simulink model "slx4"  (R2023b)
settings: Solver=ode4  StartTime=0.0  StopTime=100  FixedStep=0.01  RelTol=1e-3
values from neighbouring files (symbols this model uses):
  epsilon = sqrt((1/A_Dq)-1)    [m8.m]
  l1 = 2    [pendelPlot.m]
  l2 = 4    [pendelPlot.m]
  m1 = lsim(F1,x,t)    [m8.m]
  m2 = lsim(F2,x,t)    [m8.m]
undefined symbols (not defined in the file or in its folder): g
libraries: realtime_pacer_lib x1
settings Model: Creator=user  LastModifiedBy=user

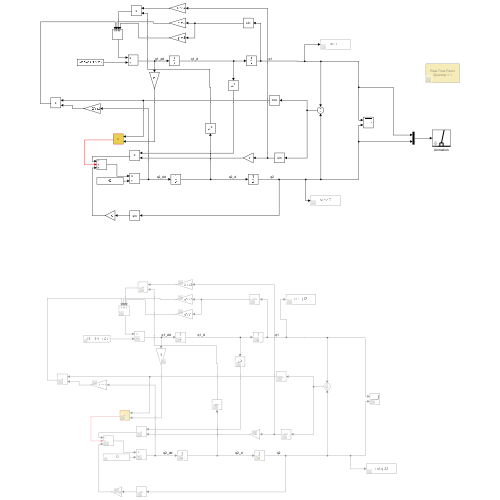
[thumbnail: Simulink's stored preview of the top-level diagram]
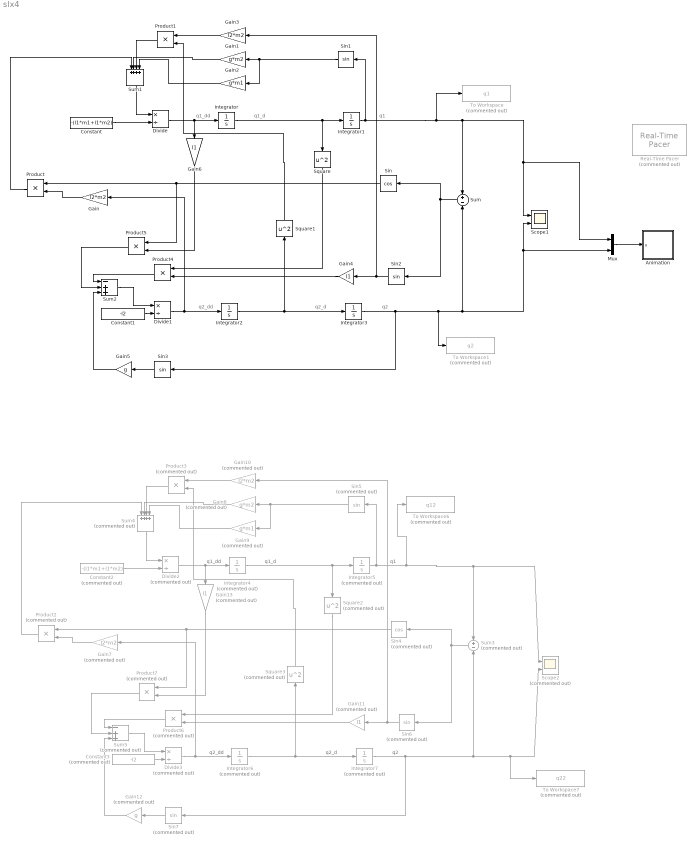
== system slx4 ==
  note: q1
  note: q1_d
  note: q1_dd
  note: q2
  note: q2_d
  note: q2_dd
  note: q1
  note: q1_d
  note: q1_dd
  note: q2
  note: q2_d
  note: q2_dd
  Animation : Subsystem  mask(Pendulum plot){}
      mask help: Pendulum plot
      mask Help: Pendulum animation function using Handle graphics.
      mask Display: plot([-10 10],[0 0],[-2 -2 2 2],[0 1 1 0],[0 3],[1 5])
  Constant : Constant  Value=-(l1*m1+l1*m2)
  Constant1 : Constant  Value=-l2
  Constant2 : Constant  Commented=on  Value=-(l1*m1+l1*m2)
  Constant3 : Constant  Commented=on  Value=-l2
  Divide : Product  Inputs=*/
  Divide1 : Product  Inputs=*/
  Divide2 : Product  Commented=on  Inputs=*/
  Divide3 : Product  Commented=on  Inputs=*/
  Gain : Gain  Gain=l2*m2
  Gain1 : Gain  Gain=g*m2
  Gain10 : Gain  Commented=on  Gain=l2*m2
  Gain11 : Gain  Commented=on  Gain=l1
  Gain12 : Gain  Commented=on  Gain=g
  Gain13 : Gain  Commented=on  Gain=l1
  Gain2 : Gain  Gain=g*m1
  Gain3 : Gain  Gain=l2*m2
  Gain4 : Gain  Gain=l1
  Gain5 : Gain  Gain=g
  Gain6 : Gain  Gain=l1
  Gain7 : Gain  Commented=on  Gain=l2*m2
  Gain8 : Gain  Commented=on  Gain=g*m2
  Gain9 : Gain  Commented=on  Gain=g*m1
  Integrator : Integrator
  Integrator1 : Integrator  InitialCondition=180/180*pi
  Integrator2 : Integrator
  Integrator3 : Integrator  InitialCondition=180/180*pi
  Integrator4 : Integrator  Commented=on
  Integrator5 : Integrator  Commented=on  InitialCondition=45/180*pi + epsilon
  Integrator6 : Integrator  Commented=on
  Integrator7 : Integrator  Commented=on  InitialCondition=180/180*pi
  Mux : Mux  Inputs=2
  Product{,1,4..5} (4 alike) : Product
  Product{2..3,6..7} (4 alike) : Product  Commented=on
  Real-Time Pacer : realtime_pacer_lib/Real-Time Pacer  Commented=on  simTimePerRealTime=1
  Scope1 : Scope  NumInputPorts=2
  Scope2 : Scope  Commented=on  NumInputPorts=2
  Sin : Trigonometry  Operator=cos
  Sin1 : Trigonometry
  Sin2 : Trigonometry
  Sin3 : Trigonometry
  Sin4 : Trigonometry  Commented=on  Operator=cos
  Sin5 : Trigonometry  Commented=on
  Sin6 : Trigonometry  Commented=on
  Sin7 : Trigonometry  Commented=on
  Square : Math  Operator=square
  Square1 : Math  Operator=square
  Square2 : Math  Commented=on  Operator=square
  Square3 : Math  Commented=on  Operator=square
  Sum : Sum  Inputs=+-
  Sum1 : Sum  Inputs=++++
  Sum2 : Sum  Inputs=-++
  Sum3 : Sum  Commented=on  Inputs=+-
  Sum4 : Sum  Commented=on  Inputs=++++
  Sum5 : Sum  Commented=on  Inputs=-++
  To Workspace : ToWorkspace  Commented=on  VariableName=q1  SampleTime=-1
  To Workspace1 : ToWorkspace  Commented=on  VariableName=q2  SampleTime=-1
  To Workspace6 : ToWorkspace  Commented=on  VariableName=q12  SampleTime=-1
  To Workspace7 : ToWorkspace  Commented=on  VariableName=q22  SampleTime=-1
  wires:
  Integrator/1 -> Integrator1/1, Square/1
  Integrator1/1 -> Sin1/1, To Workspace/1, Mux/1, Scope1/1, Sum/1
  Constant/1 -> Divide/2
  Constant1/1 -> Divide1/2
  Integrator2/1 -> Integrator3/1, Square1/1
  Divide1/1 -> Integrator2/1, Gain/1
  Sum/1 -> Sin2/1, Sin/1
  Sin/1 -> Product5/1, Product/1
  Gain/1 -> Product/2
  Product/1 -> Sum1/1
  Sum1/1 -> Divide/1
  Sin1/1 -> Gain2/1, Gain1/1
  Gain1/1 -> Sum1/2
  Gain2/1 -> Sum1/4
  Square1/1 -> Product1/2
  Integrator3/1 -> To Workspace1/1, Scope1/2, Mux/2, Sum/2, Sin3/1
  Sum2/1 -> Divide1/1
  Sin2/1 -> Gain3/1, Gain4/1
  Gain4/1 -> Product4/2
  Square/1 -> Product4/1
  Product4/1 -> Sum2/1
  Sin3/1 -> Gain5/1
  Gain5/1 -> Sum2/3
  Divide/1 -> Integrator/1, Gain6/1
  Gain6/1 -> Product5/2
  Product5/1 -> Sum2/2
  Gain3/1 -> Product1/1
  Product1/1 -> Sum1/3
  Product3/1 -> Sum4/3
  Gain10/1 -> Product3/1
  Product7/1 -> Sum5/2
  Gain13/1 -> Product7/2
  Divide2/1 -> Gain13/1, Integrator4/1
  Gain12/1 -> Sum5/3
  Sin7/1 -> Gain12/1
  Product6/1 -> Sum5/1
  Square2/1 -> Product6/1
  Gain11/1 -> Product6/2
  Sin6/1 -> Gain11/1, Gain10/1
  Sum5/1 -> Divide3/1
  Integrator7/1 -> Sin7/1, Sum3/2, Scope2/2, To Workspace7/1
  Square3/1 -> Product3/2
  Gain9/1 -> Sum4/4
  Gain8/1 -> Sum4/2
  Sin5/1 -> Gain8/1, Gain9/1
  Sum4/1 -> Divide2/1
  Product2/1 -> Sum4/1
  Gain7/1 -> Product2/2
  Sin4/1 -> Product2/1, Product7/1
  Sum3/1 -> Sin4/1, Sin6/1
  Divide3/1 -> Gain7/1, Integrator6/1
  Integrator6/1 -> Square3/1, Integrator7/1
  Constant3/1 -> Divide3/2
  Constant2/1 -> Divide2/2
  Integrator5/1 -> Sum3/1, Scope2/1, To Workspace6/1, Sin5/1
  Integrator4/1 -> Square2/1, Integrator5/1
  Mux/1 -> Animation/1(u)

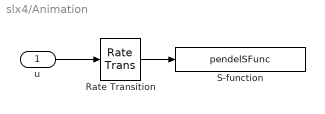
== system slx4/Animation ==
  u : Inport
  Rate Transition : RateTransition
  S-function : S-Function  FunctionName=pendelSFunc  SFunctionDeploymentMode=off  EnableBusSupport=off
      settings: DeleteFcn=pendan([],[],[],'DeleteBlock');
  wires:
  u/1 -> Rate Transition/1
  Rate Transition/1 -> S-function/1
